simulink model "test_motion_controller"  (R2023b)
settings: Solver=FixedStepAuto  StartTime=0.0  StopTime=inf  RelTol=1e-3
undefined symbols (not defined in the file): ControlModes, EstimationVelocityModes, MotionControlInitConf, SupervisorEvents
settings Model: DataDictionary=common.sldd  SimulationMode=accelerator  Creator=mfussi  LastModifiedBy=mfussi
settings SolverCC: ConcurrentTasks=on  AutoInsertRateTranBlk=on
settings DataIOCC: SaveOutput=off  DSMLogging=off  SaveTime=off  ReturnWorkspaceOutputs=off
settings OptimizationCC: UseDivisionForNetSlopeComputation=on  SimCompilerOptimization=on

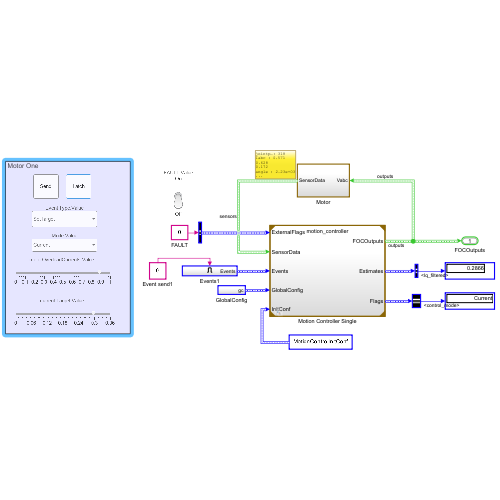
[thumbnail: Simulink's stored preview of the top-level diagram]
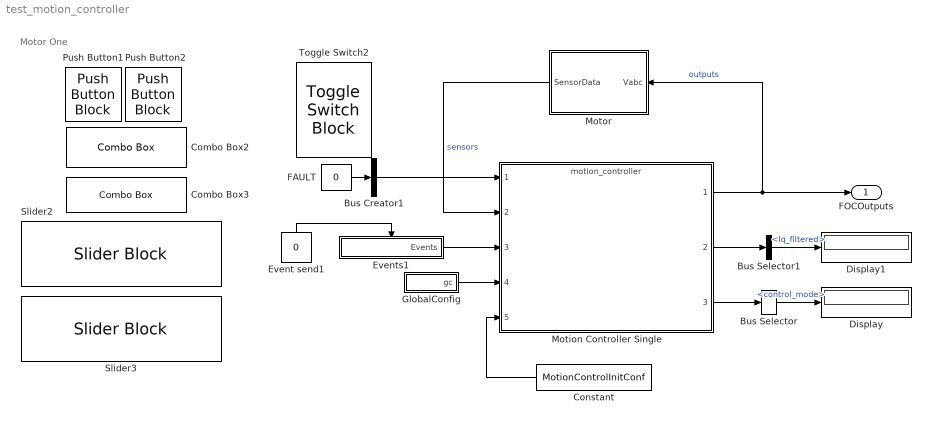
== system test_motion_controller ==
  note: Motor One
  Bus Creator1 : BusCreator  Inputs=1  OutDataTypeStr=Bus: ExternalFlags  NonVirtualBus=on
      settings: InheritFromInputs=off
  Bus Selector : BusSelector  OutputSignals=control_mode
  Bus Selector1 : BusSelector  OutputSignals=Iq_filtered
  Combo Box2 : ComboBox  SelectedLabel=SetTarget  UseEnumeratedDataType=on  EnumeratedDataType=SupervisorEvents
      settings: Values={{'None', 'SetLimit', 'SetControlMode', 'SetMotorConfig', 'SetPid', 'SetTarget'}, [0 1 2 5 3 4]}
  Combo Box3 : ComboBox  SelectedLabel=Current  UseEnumeratedDataType=on  EnumeratedDataType=ControlModes
      settings: Values={{'NotConfigured', 'Idle', 'Position', 'PositionDirect', 'Current', 'Velocity', 'Voltage', 'Torque', 'HwFaultCM'}, [0 1 2 3 4 5 6 7 8]}
  Constant : Constant  Value=MotionControlInitConf  OutDataTypeStr=Bus: ActuatorConfiguration  SampleTime=1e-3
  Display : Display
  Display1 : Display
  Event send1 : Constant  Value=0
  Events1 : Subsystem
  FAULT : Constant  Value=0  OutDataTypeStr=Inherit: Inherit via back propagation
  GlobalConfig : Subsystem
  Motion Controller Single : ModelReference  ModelNameDialog=motion_controller.slx  ModelReferenceVersion=2.190
  Motor : Subsystem
  Push Button1 : PushButtonBlock  ButtonText=Send  OffValue=0.000000
  Push Button2 : PushButtonBlock  ButtonText=Latch  ButtonType=Latch  OffValue=0.000000
  Slider2 : SliderBlock  ScaleMax=1
  Slider3 : SliderBlock  ScaleMax=0.36
  Toggle Switch2 : ToggleSwitchBlock
      settings: Values={{'Off', 'On'}, [0 1]}
  FOCOutputs : Outport  OutDataTypeStr=Bus: FOCOutputs
  wires:
  Event send1/1 -> Events1/Enable
  Bus Selector/1 -> Display/1  "<control_mode>"
  Motion Controller Single/3 -> Bus Selector/1
  Motion Controller Single/2 -> Bus Selector1/1
  Bus Creator1/1 -> Motion Controller Single/1
  Motor/1(SensorData) -> Motion Controller Single/2  "sensors"
  Motion Controller Single/1 -> Motor/1(Vabc), FOCOutputs/1  "outputs"
  Constant/1 -> Motion Controller Single/5
  Events1/1(Events) -> Motion Controller Single/3
  GlobalConfig/1(gc) -> Motion Controller Single/4
  FAULT/1 -> Bus Creator1/1
  Bus Selector1/1 -> Display1/1  "<Iq_filtered>"

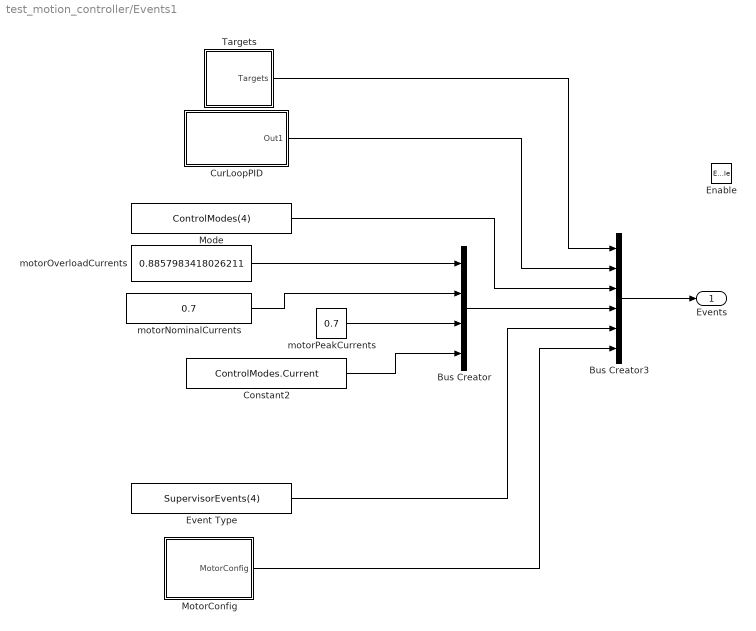
== system test_motion_controller/Events1 ==
  Enable : EnablePort
  Bus Creator : BusCreator  Inputs=4  OutDataTypeStr=Bus: SupervisorInputLimits
  Bus Creator3 : BusCreator  Inputs=6  OutDataTypeStr=Bus: SupervisorReceivedEvents  NonVirtualBus=on
      settings: InheritFromInputs=off
  Constant2 : Constant  Value=ControlModes.Current  OutDataTypeStr=Enum: ControlModes
  CurLoopPID : Subsystem  mask{OutMax=0, OutMin=0, P=2, I=500, D=0, N=10, I0=0, D0=0, shift_factor=0}
      mask prompts: shift_factor "Shift Factor"
  Event Type : Constant  Value=SupervisorEvents(4)  OutDataTypeStr=Enum: SupervisorEvents
  Mode : Constant  Value=ControlModes(4)  OutDataTypeStr=Enum: ControlModes
  MotorConfig : Subsystem
  Targets : Subsystem
  motorNominalCurrents : Constant  Value=0.7  OutDataTypeStr=single
  motorOverloadCurrents : Constant  Value=0.8857983418026211  OutDataTypeStr=single
  motorPeakCurrents : Constant  Value=0.7  OutDataTypeStr=single
  Events : Outport  OutDataTypeStr=Bus: SupervisorReceivedEvents
  wires:
  Bus Creator/1 -> Bus Creator3/4
  MotorConfig/1(MotorConfig) -> Bus Creator3/6
  Mode/1 -> Bus Creator3/3
  Targets/1(Targets) -> Bus Creator3/1
  Event Type/1 -> Bus Creator3/5
  CurLoopPID/1(Out1) -> Bus Creator3/2
  motorPeakCurrents/1 -> Bus Creator/3
  Constant2/1 -> Bus Creator/4
  motorOverloadCurrents/1 -> Bus Creator/1
  motorNominalCurrents/1 -> Bus Creator/2
  Bus Creator3/1 -> Events/1

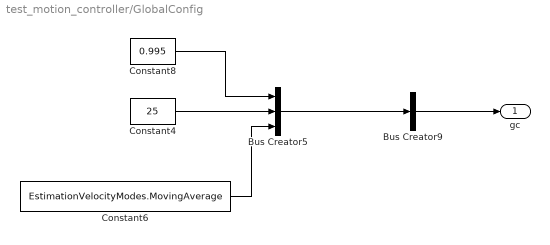
== system test_motion_controller/GlobalConfig ==
  Bus Creator5 : BusCreator  Inputs=3  OutDataTypeStr=Bus: EstimationConfiguration  NonVirtualBus=on
      settings: InheritFromInputs=off
  Bus Creator9 : BusCreator  Inputs=1  OutDataTypeStr=Bus: GlobalConfiguration  NonVirtualBus=on
      settings: InheritFromInputs=off
  Constant4 : Constant  Value=25  OutDataTypeStr=single
  Constant6 : Constant  Value=EstimationVelocityModes.MovingAverage  OutDataTypeStr=Enum: EstimationVelocityModes
  Constant8 : Constant  Value=0.995  OutDataTypeStr=single
  gc : Outport
  wires:
  Bus Creator9/1 -> gc/1
  Constant8/1 -> Bus Creator5/1
  Bus Creator5/1 -> Bus Creator9/1
  Constant4/1 -> Bus Creator5/2
  Constant6/1 -> Bus Creator5/3

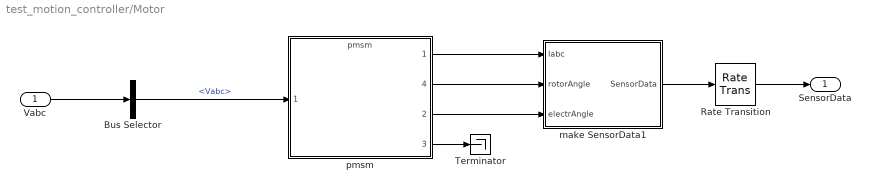
== system test_motion_controller/Motor ==
  Vabc : Inport
  Bus Selector : BusSelector  OutputSignals=Vabc
  Rate Transition : RateTransition  Integrity=off  OutPortSampleTime=ControlFOC_Ts
  Terminator : Terminator
  make SensorData1 : Subsystem
  pmsm : ModelReference  ModelNameDialog=pmsm.slx  SimulationMode=Normal  ModelReferenceVersion=7.7
      settings: PortSchema="{\"entries\":[{\"content\":{\"sides\":[{\"content\":{\"connectorIds\":[\"In1\"]},\"type\":\"ConnectorPlacement.EquallySpacedRectSide\",\"uuid\":\"210ef55b-ed00-4695-a871-354d9ae9341a\"},{\"content\":{\"connectorIds\":[\"Out1\",\"Out4\",\"Out2\",\"Out3\"],\"side\":\"RIGHT\"},\"type\":\"ConnectorPlacement.EquallySpacedRectSide\",\"uuid\":\"2c282ecd-ba90-4c60-b467-b16076ccf8b5\"},{\"content\":{\"side\":\"TOP\"},\"type\":\"ConnectorPlacement.EquallySpacedRectSide\",\"uuid\":\"fdf5a3b1-6e4d-43c2-94c4-df4906c925ba\"}]},\"type\":\"ConnectorPlacement.EquallySpacedConnector\",\"uuid\":\"b30a21c9-812d-4e38-b201-62d61a0ce6fa\"}],\"packageUris\":[\"http://schema.mathworks.com/mf0/Connector/R2020b\"],\"version\":\"1.0\"}"
  SensorData : Outport
  wires:
  make SensorData1/1(SensorData) -> Rate Transition/1
  pmsm/2 -> make SensorData1/3(electrAngle)
  pmsm/1 -> make SensorData1/1(Iabc)
  Bus Selector/1 -> pmsm/1  "<Vabc>"
  pmsm/3 -> Terminator/1
  Vabc/1 -> Bus Selector/1
  pmsm/4 -> make SensorData1/2(rotorAngle)
  Rate Transition/1 -> SensorData/1

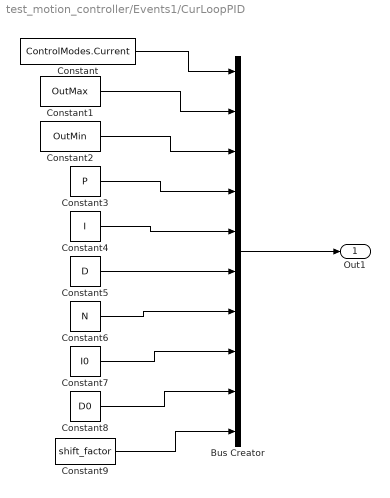
== system test_motion_controller/Events1/CurLoopPID ==
  Bus Creator : BusCreator  Inputs=10  OutDataTypeStr=Bus: PID  NonVirtualBus=on
      settings: InheritFromInputs=off
  Constant : Constant  Value=ControlModes.Current
  Constant1 : Constant  Value=OutMax  OutDataTypeStr=single
  Constant2 : Constant  Value=OutMin  OutDataTypeStr=single
  Constant3 : Constant  Value=P  OutDataTypeStr=single
  Constant4 : Constant  Value=I  OutDataTypeStr=single
  Constant5 : Constant  Value=D  OutDataTypeStr=single
  Constant6 : Constant  Value=N  OutDataTypeStr=single
  Constant7 : Constant  Value=I0  OutDataTypeStr=single
  Constant8 : Constant  Value=D0  OutDataTypeStr=single
  Constant9 : Constant  Value=shift_factor  OutDataTypeStr=uint8
  Out1 : Outport  OutDataTypeStr=Bus: PID
  wires:
  Bus Creator/1 -> Out1/1
  Constant8/1 -> Bus Creator/9
  Constant3/1 -> Bus Creator/4
  Constant5/1 -> Bus Creator/6
  Constant1/1 -> Bus Creator/2
  Constant7/1 -> Bus Creator/8
  Constant2/1 -> Bus Creator/3
  Constant9/1 -> Bus Creator/10
  Constant4/1 -> Bus Creator/5
  Constant/1 -> Bus Creator/1
  Constant6/1 -> Bus Creator/7

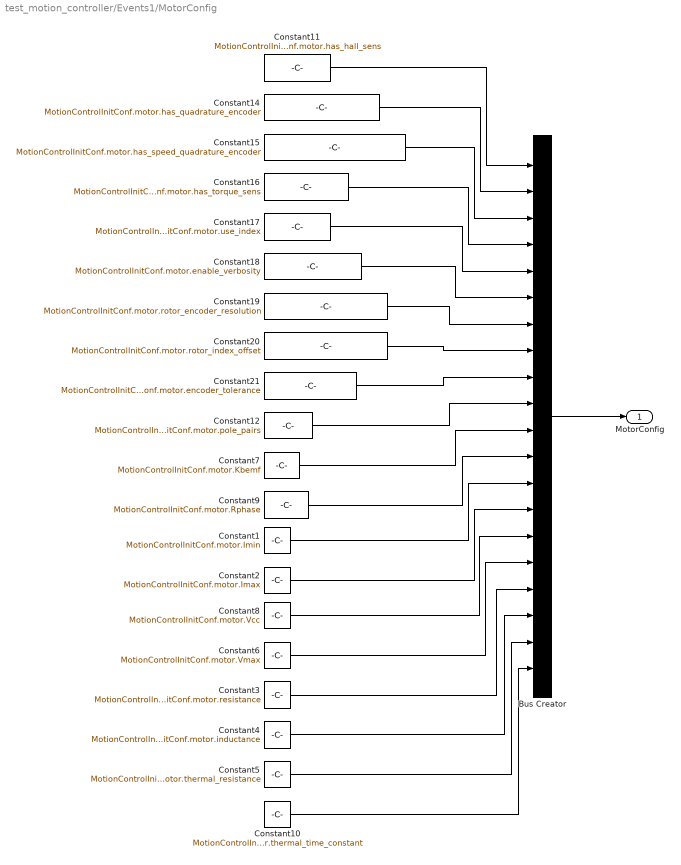
== system test_motion_controller/Events1/MotorConfig ==
  Bus Creator : BusCreator  Inputs=20  OutDataTypeStr=Bus: MotorConfiguration  NonVirtualBus=on
      settings: InheritFromInputs=off
  Constant1 : Constant  Value=MotionControlInitConf.motor.Imin  OutDataTypeStr=single
  Constant10 : Constant  Value=MotionControlInitConf.motor.thermal_time_constant  OutDataTypeStr=single
  Constant11 : Constant  Value=MotionControlInitConf.motor.has_hall_sens  OutDataTypeStr=boolean
  Constant12 : Constant  Value=MotionControlInitConf.motor.pole_pairs  OutDataTypeStr=uint8
  Constant14 : Constant  Value=MotionControlInitConf.motor.has_quadrature_encoder  OutDataTypeStr=boolean
  Constant15 : Constant  Value=MotionControlInitConf.motor.has_speed_quadrature_encoder  OutDataTypeStr=boolean
  Constant16 : Constant  Value=MotionControlInitConf.motor.has_torque_sens  OutDataTypeStr=boolean
  Constant17 : Constant  Value=MotionControlInitConf.motor.use_index  OutDataTypeStr=boolean
  Constant18 : Constant  Value=MotionControlInitConf.motor.enable_verbosity  OutDataTypeStr=boolean
  Constant19 : Constant  Value=MotionControlInitConf.motor.rotor_encoder_resolution  OutDataTypeStr=int16
  Constant2 : Constant  Value=MotionControlInitConf.motor.Imax  OutDataTypeStr=single
  Constant20 : Constant  Value=MotionControlInitConf.motor.rotor_index_offset  OutDataTypeStr=int16
  Constant21 : Constant  Value=MotionControlInitConf.motor.encoder_tolerance  OutDataTypeStr=uint8
  Constant3 : Constant  Value=MotionControlInitConf.motor.resistance  OutDataTypeStr=single
  Constant4 : Constant  Value=MotionControlInitConf.motor.inductance  OutDataTypeStr=single
  Constant5 : Constant  Value=MotionControlInitConf.motor.thermal_resistance  OutDataTypeStr=single
  Constant6 : Constant  Value=MotionControlInitConf.motor.Vmax  OutDataTypeStr=single
  Constant7 : Constant  Value=MotionControlInitConf.motor.Kbemf  OutDataTypeStr=single
  Constant8 : Constant  Value=MotionControlInitConf.motor.Vcc  OutDataTypeStr=single
  Constant9 : Constant  Value=MotionControlInitConf.motor.Rphase  OutDataTypeStr=single
  MotorConfig : Outport
  wires:
  Bus Creator/1 -> MotorConfig/1
  Constant20/1 -> Bus Creator/8
  Constant19/1 -> Bus Creator/7
  Constant21/1 -> Bus Creator/9
  Constant15/1 -> Bus Creator/3
  Constant18/1 -> Bus Creator/6
  Constant14/1 -> Bus Creator/2
  Constant16/1 -> Bus Creator/4
  Constant17/1 -> Bus Creator/5
  Constant12/1 -> Bus Creator/10
  Constant11/1 -> Bus Creator/1
  Constant7/1 -> Bus Creator/11
  Constant9/1 -> Bus Creator/12
  Constant1/1 -> Bus Creator/13
  Constant2/1 -> Bus Creator/14
  Constant8/1 -> Bus Creator/15
  Constant6/1 -> Bus Creator/16
  Constant3/1 -> Bus Creator/17
  Constant4/1 -> Bus Creator/18
  Constant5/1 -> Bus Creator/19
  Constant10/1 -> Bus Creator/20

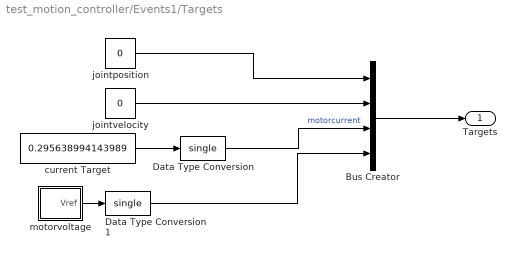
== system test_motion_controller/Events1/Targets ==
  Bus Creator : BusCreator  Inputs=4  OutDataTypeStr=Bus: Targets  NonVirtualBus=on
      settings: InheritFromInputs=off
  Data Type Conversion : DataTypeConversion  OutDataTypeStr=single  SaturateOnIntegerOverflow=off  RndMeth=Floor
  Data Type Conversion1 : DataTypeConversion  OutDataTypeStr=single  SaturateOnIntegerOverflow=off  RndMeth=Floor
  current Target : Constant  Value=0.295638994143989
  jointposition : Constant  Value=0  OutDataTypeStr=single
  jointvelocity : Constant  Value=0  OutDataTypeStr=single
  motorvoltage : Subsystem
  Targets : Outport
  wires:
  Bus Creator/1 -> Targets/1
  jointposition/1 -> Bus Creator/1
  jointvelocity/1 -> Bus Creator/2
  Data Type Conversion1/1 -> Bus Creator/4
  Data Type Conversion/1 -> Bus Creator/3  "motorcurrent"
  motorvoltage/1(Vref) -> Data Type Conversion1/1
  current Target/1 -> Data Type Conversion/1

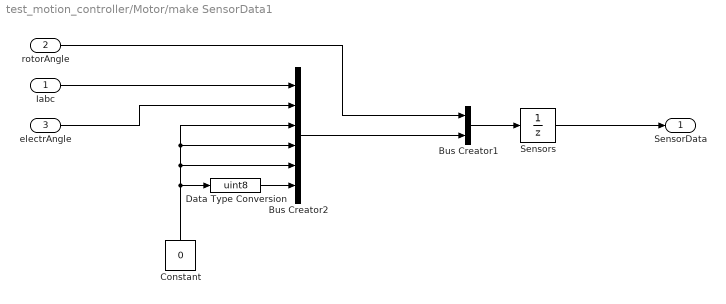
== system test_motion_controller/Motor/make SensorData1 ==
  Iabc : Inport
  rotorAngle : Inport  Port=2
  electrAngle : Inport  Port=3
  Bus Creator1 : BusCreator  Inputs=2  OutDataTypeStr=Bus: SensorsData  NonVirtualBus=on
      settings: InheritFromInputs=off
  Bus Creator2 : BusCreator  Inputs=6  OutDataTypeStr=Bus: MotorSensors  NonVirtualBus=on
      settings: InheritFromInputs=off
  Constant : Constant  Value=0  OutDataTypeStr=single
  Data Type Conversion : DataTypeConversion  OutDataTypeStr=uint8  SaturateOnIntegerOverflow=off  RndMeth=Floor
  Sensors : UnitDelay  SampleTime=-1  HasFrameUpgradeWarning=on
  SensorData : Outport
  wires:
  Sensors/1 -> SensorData/1
  Constant/1 -> Bus Creator2/4, Bus Creator2/3, Bus Creator2/5, Data Type Conversion/1
  Iabc/1 -> Bus Creator2/1
  rotorAngle/1 -> Bus Creator1/1
  Bus Creator1/1 -> Sensors/1
  electrAngle/1 -> Bus Creator2/2
  Bus Creator2/1 -> Bus Creator1/2
  Data Type Conversion/1 -> Bus Creator2/6

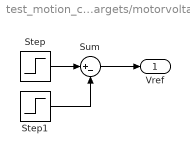
== system test_motion_controller/Events1/Targets/motorvoltage ==
  Step : Step  Time=0.1  After=100
  Step1 : Step  Time=0.2  After=60
  Sum : Sum  Inputs=|+-
  Vref : Outport
  wires:
  Sum/1 -> Vref/1
  Step1/1 -> Sum/2
  Step/1 -> Sum/1
